simulink model "QPSK_RS"  (R2017b)
settings: Solver=FixedStepAuto  StartTime=0.0  StopTime=inf  RelTol=1e-3
undefined symbols (not defined in the file): K, N, rsgenpoly
libraries: commblkcod2 x2, commdigbbndpm3 x2, commchan3 x1, commrandsrc3 x1, commsink2 x1
settings Model: Creator=phlav  LastModifiedBy=phlav
settings DataIOCC: LimitDataPoints=on  SaveOutput=off  SaveTime=off
settings OptimizationCC: BooleanDataType=off  DefaultParameterBehavior=Inlined  LocalBlockOutputs=off  LifeSpan=inf
settings DebuggingCC: AlgebraicLoopMsg=error  SingleTaskRateTransMsg=error  AllowSymbolicDim=off  SFUnexpectedBacktrackingDiag=warning  SFNoUnconditionalDefaultTransitionDiag=warning  SFExecutionAtInitializationDiag=none
settings CodeAppCC: StateflowObjectComments=on
settings GRTTargetCC: TargetLangStandard=C89/C90 (ANSI)  GeneratePreprocessorConditionals=Disable all
settings ConfigComp: CovMetricSettings=dw  CovHtmlReporting=on  CovSaveCumulativeToWorkspaceVar=on  CovSaveSingleToWorkspaceVar=on  CovExternalEMLEnable=off  CovSFcnEnable=off

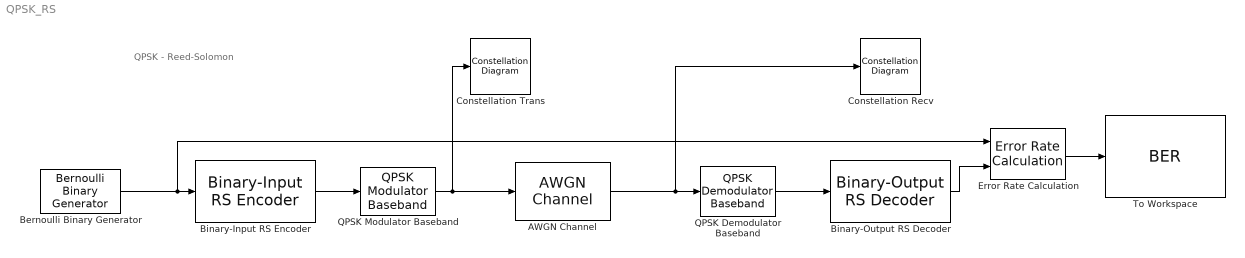
== system QPSK_RS ==
  note: QPSK - Reed-Solomon
  AWGN Channel : commchan3/AWGN Channel  InputProcessing=Columns as channels (frame based)  seed=67  noiseMode="Signal to noise ratio  (Eb/No)"  EbNodB=EbNo  EsNodB=10  SNRdB=10  bitsPerSym=2  Ps=1  Tsym=0.0002  variance=1
  Bernoulli Binary Generator : commrandsrc3/Bernoulli Binary Generator  ProbabilityOfZero=0.5  SeedSource=Auto  Seed=0  SampleTime=0.0001  SamplesPerFrame=K*ceil(log2(N+1))*10  OutputDataType=double  SimulateUsing=Interpreted execution
  Binary-Input RS Encoder : commblkcod2/Binary-Input RS Encoder  n=N  k=K  specShortening=off  shortenedK=3  specGenPoly=off  genPoly=rsgenpoly(7, 3, [], [], 'double')  specPrimPoly=off  prPoly='X^3 + X + 1'  specPuncture=off  punctVec=[ones(2,1); zeros(2,1)]  outDType=double
      settings: SourceProductName=Communications System Toolbox  SourceProductBaseCode=CM
  Binary-Output RS Decoder : commblkcod2/Binary-Output RS Decoder  n=N  k=K  specShortening=off  shortenedK=3  specGenPoly=off  genPoly=rsgenpoly(7, 3, [], [], 'double')  specPrimPoly=off  prPoly='X^3 + X + 1'  specPuncture=off  punctVec=[ones(2,1); zeros(2,1)]  specErasurePort=off  showNumErr=off  outDType=double
      settings: SourceProductName=Communications System Toolbox  SourceProductBaseCode=CM
  Constellation Recv : ConstellationDiagram
  Constellation Trans : ConstellationDiagram
  Error Rate Calculation : commsink2/Error Rate Calculation  N=0  st_delay=0  cp_mode=Entire frame  subframe=[]  PMode=Port  WsName=ErrorVec  RsMode2=off  stop=on  numErr=maxNumErrs  maxBits=maxNumBits
  QPSK Demodulator Baseband : commdigbbndpm3/QPSK Demodulator Baseband  OutType=Bit  DecType=Hard decision  VarSource=Dialog  Variance=1  Dec=Gray  Ph=pi/4  outDtype1=Inherit via internal rule  outDtype2=Inherit via internal rule  derotateFactorWordLen=16  derotateFactorDataTypeStr=Inherit: Same word length as input  derotateFactorLastDataTypeStr=Inherit: Same word length as input
  QPSK Modulator Baseband : commdigbbndpm3/QPSK Modulator Baseband  InType=Bit  Enc=Gray  Ph=pi/4  outDtype=double  outWordLen=16  outUDDataType=sfix(16)  outFracLenMode=Best precision  outFracLen=15  outDataTypeStr=double  outLastDataTypeStr=double
  To Workspace : ToWorkspace  VariableName=BER  SampleTime=-1
      settings: MaxDataPoints=1  Save2DSignal=2-D array (concatenate along first dimension)
  wires:
  Bernoulli Binary Generator/1 -> Error Rate Calculation/1, Binary-Input RS Encoder/1
  Error Rate Calculation/1 -> To Workspace/1
  QPSK Modulator Baseband/1 -> Constellation Trans/1, AWGN Channel/1
  Binary-Input RS Encoder/1 -> QPSK Modulator Baseband/1
  Binary-Output RS Decoder/1 -> Error Rate Calculation/2
  QPSK Demodulator Baseband/1 -> Binary-Output RS Decoder/1
  AWGN Channel/1 -> Constellation Recv/1, QPSK Demodulator Baseband/1
